simulink model "Lab5"  (R2021b)
settings: Solver=FixedStepAuto  StartTime=0.0  StopTime=10.0  FixedStep=50e-6  RelTol=1e-3
libraries: spsVoltageMeasurementLib x4, spsACVoltageSourceLib x3, spsCurrentMeasurementLib x3, spsRMSLib x2, spsAsynchronousMachineSIUnitsLib x1, spsDCMachineLib x1, spsDCVoltageSourceLib x1, spsGroundLib x1, spsPower3phInstantaneousLib x1, spsSeriesRLCBranchLib x1, spspowerguiLib x1
settings Model: Creator=coolk  LastModifiedBy=coolk

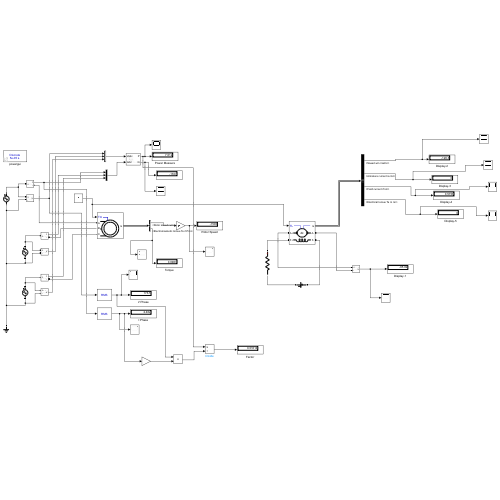
[thumbnail: Simulink's stored preview of the top-level diagram]
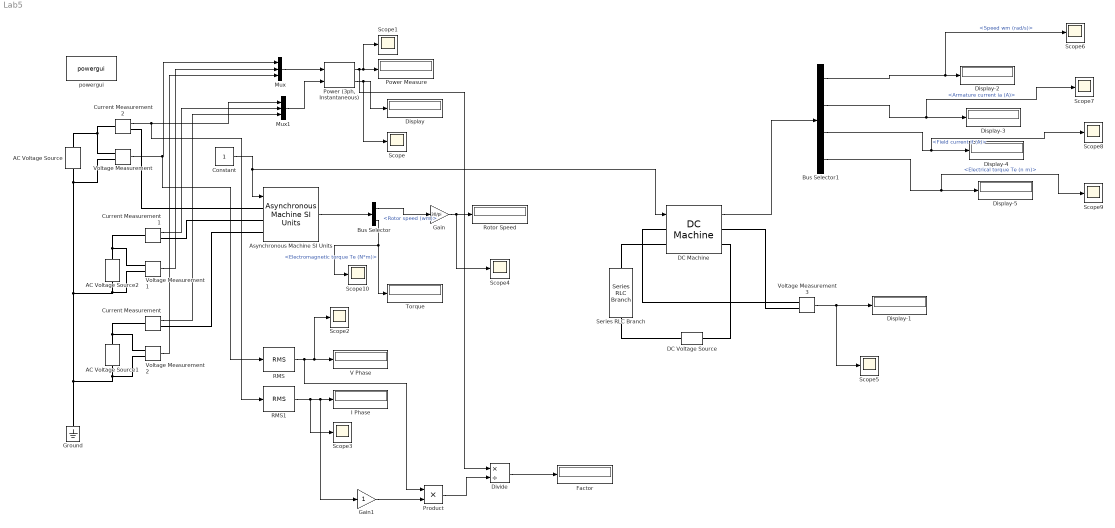
== system Lab5 ==
  AC Voltage Source : spsACVoltageSourceLib/AC Voltage Source  Amplitude=239.600362  Phase=0  Frequency=50  SampleTime=0  Measurements=None  BusType=swing  Pref=10e3  Qref=0  Qmin=-inf  Qmax=+inf
  AC Voltage Source1 : spsACVoltageSourceLib/AC Voltage Source  Amplitude=239.600362  Phase=240  Frequency=50  SampleTime=0  Measurements=None  BusType=swing  Pref=10e3  Qref=0  Qmin=-inf  Qmax=+inf
  AC Voltage Source2 : spsACVoltageSourceLib/AC Voltage Source  Amplitude=239.600362  Phase=120  Frequency=50  SampleTime=0  Measurements=None  BusType=swing  Pref=10e3  Qref=0  Qmin=-inf  Qmax=+inf
  Asynchronous Machine SI Units : spsAsynchronousMachineSIUnitsLib/Asynchronous Machine SI Units  RotorType=Squirrel-cage  PresetModel="01:  5 HP   460 V 60Hz 1750 RPM"  MechanicalLoad=Torque Tm  ShowDetailedParameters=on  ReferenceFrame=Rotor  Units=SI  MeasurementBus=off  NominalParameters=[3730 460 60]  VoltageRatio=1  Stator=[1.115 0.005974]  Rotor=[1.083 0.005974]  Cage1=[0.4155 0.002066]  Cage2=[0.4168 0.0003495]  Lm=0.2037  Mechanical=[0.02 0.005752 2]  PolePairs=2  InitialConditions=[0 0 0 0 0 0 0 0]  SimulateSaturation=off  Saturation=[14.03593122, 27.81365428, 53.79336849, 72.68890987, 97.98006896, 148.6815601, 215.7428561, 302.9841135, 428.7778367 ; 230, 322, 414, 460, 506, 552, 598, 644, 690]  LoadFlowParameters=1492000  TsPowergui=0  TsBlock=-1  IterativeModel=Trapezoidal non iterative  IterativeDiscreteModel=Trapezoidal non iterative  Pmec=1.492e+006
  Bus Selector : BusSelector  OutputSignals=Mechanical.Rotor speed (wm),Mechanical.Electromagnetic torque Te (N*m)
  Bus Selector1 : BusSelector  OutputSignals=Speed wm (rad/s),Armature current ia (A),Field current if (A),Electrical torque Te (n m)
  Constant : Constant
  Current Measurement : spsCurrentMeasurementLib/Current Measurement  PhasorSimulation=off  OutputType=Complex  PSBequivalent=0
  Current Measurement1 : spsCurrentMeasurementLib/Current Measurement  PhasorSimulation=off  OutputType=Complex  PSBequivalent=0
  Current Measurement2 : spsCurrentMeasurementLib/Current Measurement  PhasorSimulation=off  OutputType=Complex  PSBequivalent=0
  DC Machine : spsDCMachineLib/DC Machine  PresetModel=01: 5HP 240V 1750RPM Field:300V  MechanicalLoad=Torque TL  FieldType=Wound  ShowDetailedParameters=on  MeasurementBus=off  RLa=[2.581 0.028]  RLf=[281.2 156]  Laf=0.9483  MachineConstant=Torque constant (N.m/A)  Ke=1.8  Kt=1.8  J=0.02215  Bm=0.002953  Tf=0.5161  w0=1  Ifinit=0.575594781273983  TsPowergui=0  TsBlock=-1
  DC Voltage Source : spsDCVoltageSourceLib/DC Voltage Source  Amplitude=300  Measurements=None
  Display : Display
  Display-{1..5} (5 alike) : Display
  Divide : Product  Inputs=*/
  Factor : Display
  Gain : Gain  Gain=30/pi
  Gain1 : Gain
  Ground : spsGroundLib/Ground  LConnTagsString=a
  I Phase : Display
  Mux : Mux  Inputs=3
  Mux1 : Mux  Inputs=3
  "Power (3ph, Instantaneous)" : spsPower3phInstantaneousLib/Power (3ph, Instantaneous)
  Power Measure : Display
  Product : Product
  RMS : spsRMSLib/RMS  TrueRMS=on  Freq=60  RMSInit=120  Ts=50e-6
  RMS1 : spsRMSLib/RMS  TrueRMS=on  Freq=60  RMSInit=120  Ts=50e-6
  Rotor Speed : Display
  Scope{,1..10} (11 alike) : Scope
  Series RLC Branch : spsSeriesRLCBranchLib/Series RLC Branch  LConnTagsString=__new0  RConnTagsString=__new0  BranchType=R  Resistance=240  Inductance=0  SetiL0=off  InitialCurrent=0  Capacitance=0  Setx0=off  InitialVoltage=0  Measurements=None
  Torque : Display
  V Phase : Display
  Voltage Measurement{,1..3} (4 alike) : spsVoltageMeasurementLib/Voltage Measurement  PhasorSimulation=off  OutputType=Complex  PSBequivalent=0
  powergui : spspowerguiLib/powergui  Priority=1  SimulationMode=Discrete  SampleTime=50e-6  frequency=60  Iterations=50  frequencyindice=0  Pbase=100e6  ErrMax=1e-4  UnitsV=kV  UnitsW=MW  buscounter=0  FunctionMessages=off  echomessages=off  EnableUseOfTLC=off  CurrentSourceSwitches=off  DisableSnubberDevices=off  DisableRonSwitches=off  DisableVfSwitches=off  DisplayEquations=off  AutomaticDiscreteSolvers=off  SolverType=Tustin/Backward Euler (TBE)  Interpol=off  ExternalGateDelay=off  methode=off  Ts=100  x0status=blocks  SPID=on  SwTol=0  HookPort=off  NonlinearTolerance=1e-4  nMaxIteration=100  ContinueOnMaxIteration=off  RestoreLinks=warning  ResistiveCurrentMeasurement=off  Frange=[0:2:500]  Ylog=off  Xlog=on  ShowGrid=off  save=off  variable=ZData  structure=0  ZoomFFT=off  StartTime=0.0  cycles=1  DisplayStyle=1  fundamental=60  FreqAxis=off  MaxFrequency=1000  frequencyindicesteady=1  RmsSteady=1  display=off
  wires:
  Gain/1 -> Scope4/1, Rotor Speed/1
  Current Measurement1/1 -> Mux1/2
  RMS1/1 -> Scope3/1, Gain1/1, I Phase/1
  Bus Selector/1 -> Gain/1  "<Rotor speed (wm)>"
  Asynchronous Machine SI Units/1 -> Bus Selector/1
  "Power (3ph, Instantaneous)"/2 -> Display/1, Scope/1
  Mux/1 -> "Power (3ph, Instantaneous)"/1
  Voltage Measurement/1 -> RMS/1, Mux/1
  Mux1/1 -> "Power (3ph, Instantaneous)"/2
  Voltage Measurement1/1 -> Mux/2
  "Power (3ph, Instantaneous)"/1 -> Divide/1, Scope1/1, Power Measure/1
  Current Measurement/1 -> Mux1/3
  Current Measurement2/1 -> RMS1/1, Mux1/1
  RMS/1 -> Product/1, Scope2/1, V Phase/1
  Voltage Measurement2/1 -> Mux/3
  Constant/1 -> DC Machine/1, Asynchronous Machine SI Units/1
  Gain1/1 -> Product/2
  Product/1 -> Divide/2
  Divide/1 -> Factor/1
  Voltage Measurement3/1 -> Scope5/1, Display-1/1
  DC Machine/1 -> Bus Selector1/1
  Bus Selector1/1 -> Scope6/1, Display-2/1  "<Speed wm (rad/s)>"
  Bus Selector1/2 -> Scope7/1, Display-3/1  "<Armature current ia (A)>"
  Bus Selector1/3 -> Scope8/1, Display-4/1  "<Field current if (A)>"
  Bus Selector1/4 -> Scope9/1, Display-5/1  "<Electrical torque Te (n m)>"
  Bus Selector/2 -> Scope10/1, Torque/1  "<Electromagnetic torque Te (N*m)>"
  connections:
  AC Voltage Source1/RConn1 -- Voltage Measurement2/LConn1 -- Current Measurement/LConn1
  AC Voltage Source/RConn1 -- Voltage Measurement/LConn1 -- Current Measurement2/LConn1
  Current Measurement1/LConn1 -- Voltage Measurement1/LConn1 -- AC Voltage Source2/RConn1
  Ground/LConn1 -- AC Voltage Source/LConn1 -- Voltage Measurement/LConn2 -- Voltage Measurement1/LConn2 -- AC Voltage Source2/LConn1 -- Voltage Measurement2/LConn2 -- AC Voltage Source1/LConn1
  Current Measurement/RConn1 -- Asynchronous Machine SI Units/LConn3
  Current Measurement2/RConn1 -- Asynchronous Machine SI Units/LConn1
  Current Measurement1/RConn1 -- Asynchronous Machine SI Units/LConn2
  DC Voltage Source/LConn1 -- DC Machine/RConn2
  DC Machine/RConn1 -- Voltage Measurement3/LConn2
  DC Machine/LConn1 -- Voltage Measurement3/LConn1
  DC Machine/LConn2 -- Series RLC Branch/LConn1
  Series RLC Branch/RConn1 -- DC Voltage Source/RConn1
